simulink model "LFC_NN"  (Simulink 7.8)
settings: Solver=ode8  StartTime=0.0  StopTime=60  FixedStep=0.01  RelTol=1e-3
values from neighbouring files (symbols this model uses):
  DPd1 = In(2)    [AREA1.m]    (also in Main.m = 0.3)
  DPd2 = In(2)    [AREA2.m]    (also in Main.m = 0.1)
  DPd3 = In(2)    [AREA3.m]    (also in Main.m = 0.01)
settings Model: Creator=Mahdi  LastModifiedBy=Mahdi

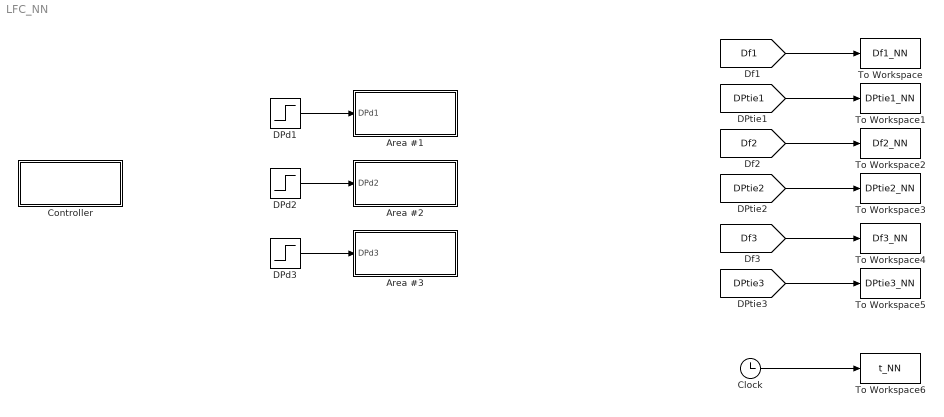
== system LFC_NN ==
  Area #1 : Subsystem
  Area #2 : Subsystem
  Area #3 : Subsystem
  Clock : Clock
  Controller : Subsystem
  DPd1 : Step  Time=0  After=DPd1  SampleTime=0
  DPd2 : Step  Time=0  After=DPd2  SampleTime=0
  DPd3 : Step  Time=0  After=DPd3  SampleTime=0
  To Workspace : ToWorkspace  VariableName=Df1_NN  SampleTime=-1  SaveFormat=Array
  To Workspace1 : ToWorkspace  VariableName=DPtie1_NN  SampleTime=-1  SaveFormat=Array
  To Workspace2 : ToWorkspace  VariableName=Df2_NN  SampleTime=-1  SaveFormat=Array
  To Workspace3 : ToWorkspace  VariableName=DPtie2_NN  SampleTime=-1  SaveFormat=Array
  To Workspace4 : ToWorkspace  VariableName=Df3_NN  SampleTime=-1  SaveFormat=Array
  To Workspace5 : ToWorkspace  VariableName=DPtie3_NN  SampleTime=-1  SaveFormat=Array
  To Workspace6 : ToWorkspace  VariableName=t_NN  SampleTime=-1  SaveFormat=Array
  wires:
  DPd1/1 -> Area #1/1(DPd1)
  DPd2/1 -> Area #2/1(DPd2)
  DPd3/1 -> Area #3/1(DPd3)
  [Df1] -> To Workspace/1
  [DPtie1] -> To Workspace1/1
  [Df2] -> To Workspace2/1
  [DPtie2] -> To Workspace3/1
  [Df3] -> To Workspace4/1
  [DPtie3] -> To Workspace5/1
  Clock/1 -> To Workspace6/1

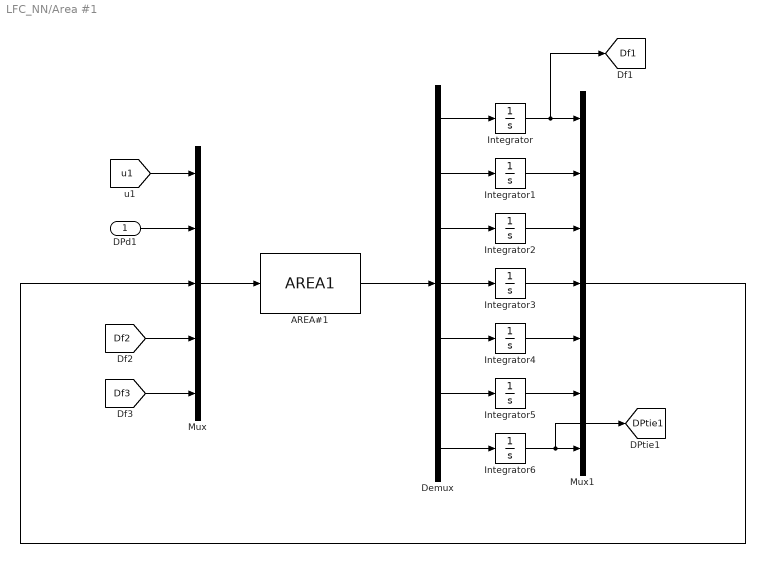
== system LFC_NN/Area #1 ==
  DPd1 : Inport
  AREA#1 : MATLABFcn  MATLABFcn=AREA1
  Demux : Demux  Outputs=7
  Integrator{,1..6} (7 alike) : Integrator
  Mux : Mux  Inputs=5
  Mux1 : Mux  Inputs=7
  tag scope: DPtie1=global, Df1=global
  wires:
  AREA#1/1 -> Demux/1
  Mux/1 -> AREA#1/1
  Demux/1 -> Integrator/1
  Demux/2 -> Integrator1/1
  Demux/3 -> Integrator2/1
  Demux/4 -> Integrator3/1
  Demux/5 -> Integrator4/1
  Demux/6 -> Integrator5/1
  Demux/7 -> Integrator6/1
  Integrator/1 -> Mux1/1, [Df1]
  Integrator1/1 -> Mux1/2
  Integrator2/1 -> Mux1/3
  Integrator3/1 -> Mux1/4
  Integrator4/1 -> Mux1/5
  Integrator6/1 -> Mux1/7, [DPtie1]
  Integrator5/1 -> Mux1/6
  [u1] -> Mux/1
  DPd1/1 -> Mux/2
  [Df2] -> Mux/4
  [Df3] -> Mux/5
  Mux1/1 -> Mux/3

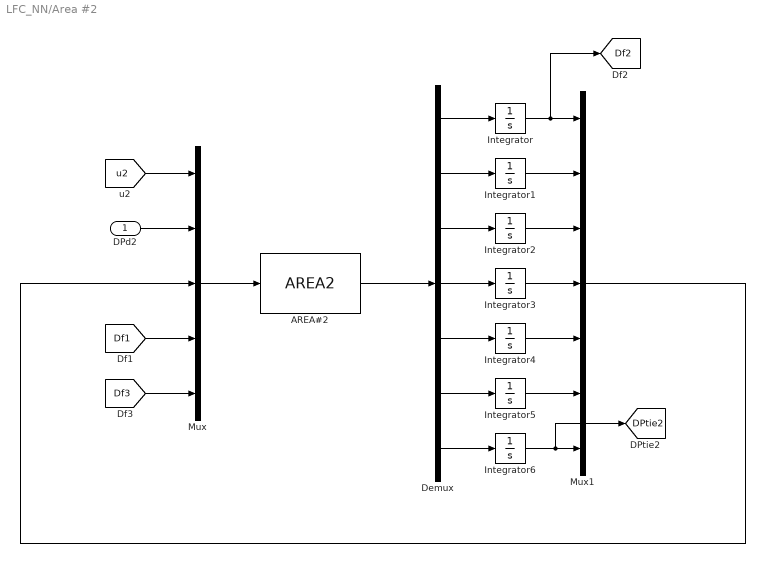
== system LFC_NN/Area #2 ==
  DPd2 : Inport
  AREA#2 : MATLABFcn  MATLABFcn=AREA2
  Demux : Demux  Outputs=7
  Integrator{,1..6} (7 alike) : Integrator
  Mux : Mux  Inputs=5
  Mux1 : Mux  Inputs=7
  tag scope: DPtie2=global, Df2=global
  wires:
  AREA#2/1 -> Demux/1
  Mux/1 -> AREA#2/1
  Demux/1 -> Integrator/1
  Demux/2 -> Integrator1/1
  Demux/3 -> Integrator2/1
  Demux/4 -> Integrator3/1
  Demux/5 -> Integrator4/1
  Demux/6 -> Integrator5/1
  Demux/7 -> Integrator6/1
  Integrator/1 -> Mux1/1, [Df2]
  Integrator1/1 -> Mux1/2
  Integrator2/1 -> Mux1/3
  Integrator3/1 -> Mux1/4
  Integrator4/1 -> Mux1/5
  Integrator6/1 -> Mux1/7, [DPtie2]
  Integrator5/1 -> Mux1/6
  Mux1/1 -> Mux/3
  [u2] -> Mux/1
  DPd2/1 -> Mux/2
  [Df1] -> Mux/4
  [Df3] -> Mux/5

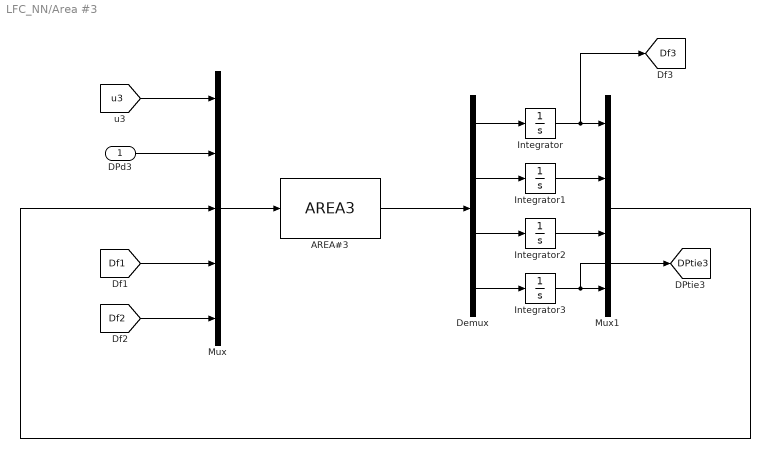
== system LFC_NN/Area #3 ==
  DPd3 : Inport
  AREA#3 : MATLABFcn  MATLABFcn=AREA3
  Demux : Demux
  Integrator{,1..3} (4 alike) : Integrator
  Mux : Mux  Inputs=5
  Mux1 : Mux
  tag scope: DPtie3=global, Df3=global
  wires:
  Demux/1 -> Integrator/1
  Demux/2 -> Integrator1/1
  Demux/3 -> Integrator2/1
  Demux/4 -> Integrator3/1
  Integrator/1 -> Mux1/1, [Df3]
  Integrator1/1 -> Mux1/2
  Integrator2/1 -> Mux1/3
  Integrator3/1 -> Mux1/4, [DPtie3]
  AREA#3/1 -> Demux/1
  Mux/1 -> AREA#3/1
  [u3] -> Mux/1
  DPd3/1 -> Mux/2
  [Df1] -> Mux/4
  [Df2] -> Mux/5
  Mux1/1 -> Mux/3

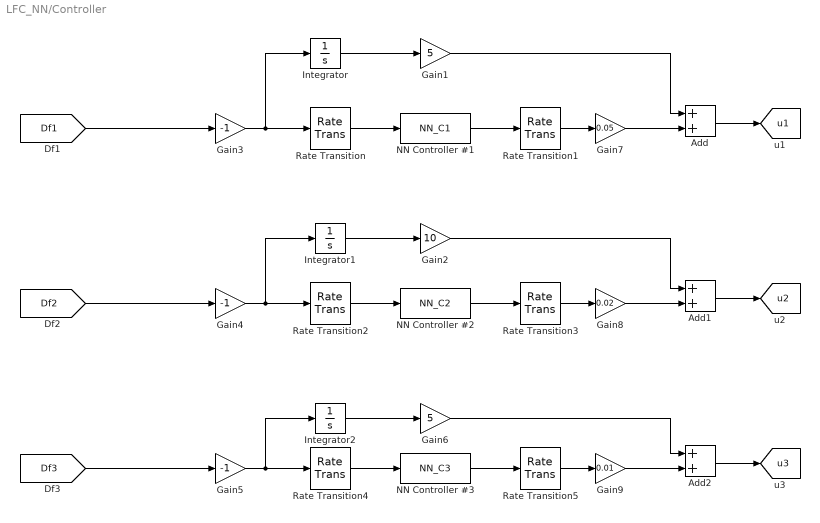
== system LFC_NN/Controller ==
  Add : Sum
  Add1 : Sum
  Add2 : Sum
  Gain1 : Gain  Gain=5
  Gain2 : Gain  Gain=10
  Gain3 : Gain  Gain=-1
  Gain4 : Gain  Gain=-1
  Gain5 : Gain  Gain=-1
  Gain6 : Gain  Gain=5
  Gain7 : Gain  Gain=0.05
  Gain8 : Gain  Gain=0.02
  Gain9 : Gain  Gain=0.01
  Integrator : Integrator
  Integrator1 : Integrator
  Integrator2 : Integrator
  NN Controller #1 : MATLABFcn  MATLABFcn=NN_C1  SampleTime=0.1
  NN Controller #2 : MATLABFcn  MATLABFcn=NN_C2  SampleTime=0.1
  NN Controller #3 : MATLABFcn  MATLABFcn=NN_C3  SampleTime=0.1
  Rate Transition : RateTransition  OutPortSampleTime=0.1
  Rate Transition1 : RateTransition
  Rate Transition2 : RateTransition  OutPortSampleTime=0.1
  Rate Transition3 : RateTransition
  Rate Transition4 : RateTransition  OutPortSampleTime=0.1
  Rate Transition5 : RateTransition
  tag scope: u1=global, u2=global, u3=global
  wires:
  [Df1] -> Gain3/1
  [Df2] -> Gain4/1
  [Df3] -> Gain5/1
  Gain3/1 -> Rate Transition/1, Integrator/1
  NN Controller #1/1 -> Rate Transition1/1
  Rate Transition/1 -> NN Controller #1/1
  NN Controller #2/1 -> Rate Transition3/1
  Rate Transition2/1 -> NN Controller #2/1
  Gain4/1 -> Rate Transition2/1, Integrator1/1
  NN Controller #3/1 -> Rate Transition5/1
  Rate Transition4/1 -> NN Controller #3/1
  Gain5/1 -> Rate Transition4/1, Integrator2/1
  Integrator/1 -> Gain1/1
  Integrator1/1 -> Gain2/1
  Integrator2/1 -> Gain6/1
  Rate Transition1/1 -> Gain7/1
  Gain1/1 -> Add/1
  Add/1 -> [u1]
  Rate Transition3/1 -> Gain8/1
  Gain2/1 -> Add1/1
  Add1/1 -> [u2]
  Rate Transition5/1 -> Gain9/1
  Gain6/1 -> Add2/1
  Add2/1 -> [u3]
  Gain7/1 -> Add/2
  Gain8/1 -> Add1/2
  Gain9/1 -> Add2/2
